simulink model "DOC_O2_ECU"  (R2019a)
settings: Solver=VariableStepAuto  StartTime=0.0  StopTime=10.0  RelTol=1e-3
undefined symbols (not defined in the file or in its folder): O2
libraries: simulink x3
settings Model: Creator=Home  LastModifiedBy=User
settings DataIOCC: ReturnWorkspaceOutputs=off
settings DebuggingCC: PregeneratedLibrarySubsystemCodeDiagnostic=none  ArithmeticOperatorsInVariantConditions=warning
settings SFSimCC: SimUseLocalCustomCode=off
settings RTWCC: RTWUseLocalCustomCode=off

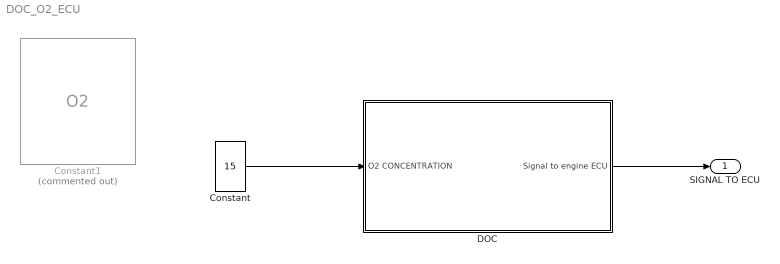
== system DOC_O2_ECU ==
  Constant : Constant  Value=15
  Constant1 : Constant  Commented=on  Value=O2
  DOC : Subsystem
  SIGNAL TO ECU : Outport
  wires:
  Constant/1 -> DOC/1(O2 CONCENTRATION)
  DOC/1(Signal to engine ECU) -> SIGNAL TO ECU/1

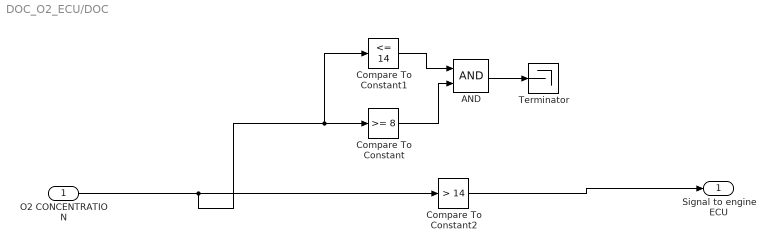
== system DOC_O2_ECU/DOC ==
  O2 CONCENTRATION : Inport
  AND : Logic  AllPortsSameDT=off  OutDataTypeStr=boolean
  Compare To Constant : simulink/Logic and Bit Operations/Compare To Constant  relop=>=  const=8  OutDataTypeStr=boolean
  Compare To Constant1 : simulink/Logic and Bit Operations/Compare To Constant  relop=<=  const=14  OutDataTypeStr=boolean
  Compare To Constant2 : simulink/Logic and Bit Operations/Compare To Constant  relop=>  const=14  OutDataTypeStr=boolean
  Terminator : Terminator
  Signal to engine ECU : Outport
  wires:
  Compare To Constant2/1 -> Signal to engine ECU/1
  O2 CONCENTRATION/1 -> Compare To Constant1/1, Compare To Constant/1, Compare To Constant2/1
  Compare To Constant1/1 -> AND/1
  Compare To Constant/1 -> AND/2
  AND/1 -> Terminator/1
